simulink model "ENV_NEW"  (R2024b)
settings: Solver=FixedStepDiscrete  StartTime=0.0  StopTime=1  FixedStep=0.001  RelTol=1e-3  EnableMultiTasking=on
libraries: stm32blockslib x105, canmsglib x32, stm32f4xxblockslib x11, simulink x10
(part 5 of 5)

== matlab function ENV_NEW/CAN RX2/Enabled Subsystem/MATLAB Function7 ==
  data: RxBytes input uint8 size=15; Message output Bus: CANMessage
function Message = DecodeCANMsg(RxBytes)
%#codegen
% RxBytes is uint8(1x15); bytes 1-2 are don't-care (command echo + one turnaround byte)
SIDH = RxBytes(3);
SIDL = RxBytes(4);
EID8 = RxBytes(5);
EID0 = RxBytes(6);
DLC  = RxBytes(7);

Message.ID       = uint32(bitor(uint32(bitshift(uint32(SIDH), 3)), ...
                        uint32(bitshift(uint32(SIDL), -5))));
Message.Extended = false;
Message.Remote   = false;
Message.Error    = false;
Message.Length   = double(bitand(DLC, uint8(15)));
Message.Data     = RxBytes(8:15);

== matlab function ENV_NEW/CAN RX3/Enabled Subsystem/MATLAB Function7 ==
  data: RxBytes input uint8 size=15; Message output Bus: CANMessage
function Message = DecodeCANMsg(RxBytes)
%#codegen
% RxBytes is uint8(1x15); bytes 1-2 are don't-care (command echo + one turnaround byte)
SIDH = RxBytes(3);
SIDL = RxBytes(4);
EID8 = RxBytes(5);
EID0 = RxBytes(6);
DLC  = RxBytes(7);

Message.ID       = uint32(bitor(uint32(bitshift(uint32(SIDH), 3)), ...
                        uint32(bitshift(uint32(SIDL), -5))));
Message.Extended = false;
Message.Remote   = false;
Message.Error    = false;
Message.Length   = double(bitand(DLC, uint8(15)));
Message.Data     = RxBytes(8:15);

== matlab function ENV_NEW/CAN Tx/MATLAB Function2 ==
  settings: updateMethod=DISCRETE  sampleTime=.001
  data: WriteInstruction output; ID input uint32; CANVector output uint8; Length input uint8; Data input uint8; RTS input; RTSByte output; period input; offset input; MCPInitialized input
function [WriteInstruction, CANVector, RTSByte] = ConvertToVector(ID, Length, Data, RTS, period, offset, MCPInitialized)
%#codegen
persistent count;
if isempty(count)
    count = uint16(0);
end

if MCPInitialized
    if count == uint16(offset)
        id_u16 = uint16(ID);
        CANVector = zeros(1,13,'uint8');
        CANVector(1) = uint8(bitshift(id_u16, -3));
        CANVector(2) = uint8(bitshift(bitand(id_u16, uint16(7)), 5));
        CANVector(3) = uint8(0);
        CANVector(4) = uint8(0);
        CANVector(5) = bitand(uint8(Length), uint8(15));
        for i = 1:8
            CANVector(5+i) = uint8(Data(i));
        end
        RTSByte = uint8(RTS);
        WriteInstruction = uint8(0x02);
    else
        CANVector = zeros(1,13,'uint8');
        RTSByte = uint8(RTS);
        WriteInstruction = uint8(0x03);
    end

    count = count + uint16(1);
    if count >= uint16(period)
        count = uint16(0);
    end
else
    CANVector = zeros(1,13,'uint8');
    RTSByte = uint8(0x03);
    WriteInstruction = uint8(0x03);
    % don't increment count while MCP not ready
end

== matlab function ENV_NEW/CAN Tx/MATLAB Function4 ==
  settings: updateMethod=DISCRETE  sampleTime=.001
  data: WriteInstruction output; ID input uint32; CANVector output uint8; Length input uint8; Data input uint8; RTS input; RTSByte output; period input; offset input; MCPInitialized input
function [WriteInstruction, CANVector, RTSByte] = ConvertToVector(ID, Length, Data, RTS, period, offset, MCPInitialized)
%#codegen
persistent count;
if isempty(count)
    count = uint16(0);
end

if MCPInitialized
    if count == uint16(offset)
        id_u16 = uint16(ID);
        CANVector = zeros(1,13,'uint8');
        CANVector(1) = uint8(bitshift(id_u16, -3));
        CANVector(2) = uint8(bitshift(bitand(id_u16, uint16(7)), 5));
        CANVector(3) = uint8(0);
        CANVector(4) = uint8(0);
        CANVector(5) = bitand(uint8(Length), uint8(15));
        for i = 1:8
            CANVector(5+i) = uint8(Data(i));
        end
        RTSByte = uint8(RTS);
        WriteInstruction = uint8(0x02);
    else
        CANVector = zeros(1,13,'uint8');
        RTSByte = uint8(RTS);
        WriteInstruction = uint8(0x03);
    end

    count = count + uint16(1);
    if count >= uint16(period)
        count = uint16(0);
    end
else
    CANVector = zeros(1,13,'uint8');
    RTSByte = uint8(0x03);
    WriteInstruction = uint8(0x03);
    % don't increment count while MCP not ready
end

== matlab function ENV_NEW/CAN3 RX/MATLAB Function3 ==
  data: RxBytes input uint8 size=15; Message output Bus: CANMessage
function Message = DecodeCANMsg(RxBytes)
%#codegen
% RxBytes is uint8(1x15); bytes 1-2 are don't-care (command echo + one turnaround byte)
SIDH = RxBytes(3);
SIDL = RxBytes(4);
EID8 = RxBytes(5);
EID0 = RxBytes(6);
DLC  = RxBytes(7);

Message.ID       = uint32(bitor(uint32(bitshift(uint32(SIDH), 3)), ...
                        uint32(bitshift(uint32(SIDL), -5))));
Message.Extended = false;
Message.Remote   = false;
Message.Error    = false;
Message.Length   = double(bitand(DLC, uint8(15)));
Message.Data     = RxBytes(8:15);

== matlab function ENV_NEW/CAN3 RX/MATLAB Function4 ==
  data: RxBytes input uint8 size=15; Message output Bus: CANMessage
function Message = DecodeCANMsg(RxBytes)
%#codegen
% RxBytes is uint8(1x15); bytes 1-2 are don't-care (command echo + one turnaround byte)
SIDH = RxBytes(3);
SIDL = RxBytes(4);
EID8 = RxBytes(5);
EID0 = RxBytes(6);
DLC  = RxBytes(7);

Message.ID       = uint32(bitor(uint32(bitshift(uint32(SIDH), 3)), ...
                        uint32(bitshift(uint32(SIDL), -5))));
Message.Extended = false;
Message.Remote   = false;
Message.Error    = false;
Message.Length   = double(bitand(DLC, uint8(15)));
Message.Data     = RxBytes(8:15);

== matlab function ENV_NEW/CAN3 RX/MATLAB Function5 ==
  data: RxBytes input uint8 size=15; Message output Bus: CANMessage
function Message = DecodeCANMsg(RxBytes)
%#codegen
% RxBytes is uint8(1x15); bytes 1-2 are don't-care (command echo + one turnaround byte)
SIDH = RxBytes(3);
SIDL = RxBytes(4);
EID8 = RxBytes(5);
EID0 = RxBytes(6);
DLC  = RxBytes(7);

Message.ID       = uint32(bitor(uint32(bitshift(uint32(SIDH), 3)), ...
                        uint32(bitshift(uint32(SIDL), -5))));
Message.Extended = false;
Message.Remote   = false;
Message.Error    = false;
Message.Length   = double(bitand(DLC, uint8(15)));
Message.Data     = RxBytes(8:15);

== matlab function ENV_NEW/CAN3 RX/MATLAB Function6 ==
  data: RxBytes input uint8 size=15; Message output Bus: CANMessage
function Message = DecodeCANMsg(RxBytes)
%#codegen
% RxBytes is uint8(1x15); bytes 1-2 are don't-care (command echo + one turnaround byte)
SIDH = RxBytes(3);
SIDL = RxBytes(4);
EID8 = RxBytes(5);
EID0 = RxBytes(6);
DLC  = RxBytes(7);

Message.ID       = uint32(bitor(uint32(bitshift(uint32(SIDH), 3)), ...
                        uint32(bitshift(uint32(SIDL), -5))));
Message.Extended = false;
Message.Remote   = false;
Message.Error    = false;
Message.Length   = double(bitand(DLC, uint8(15)));
Message.Data     = RxBytes(8:15);
